simulink model "SpringModel"  (R2018a)
settings: Solver=ode45  StartTime=0.0  StopTime=1  MaxStep=1e-4  MinStep=1e-6  RelTol=1e-4  AbsTol=1e-7
settings Model: Creator=thoma_000  LastModifiedBy=thoma_000
settings SolverCC: ZeroCrossAlgorithm=Adaptive
settings DebuggingCC: MaxConsecutiveZCsMsg=none

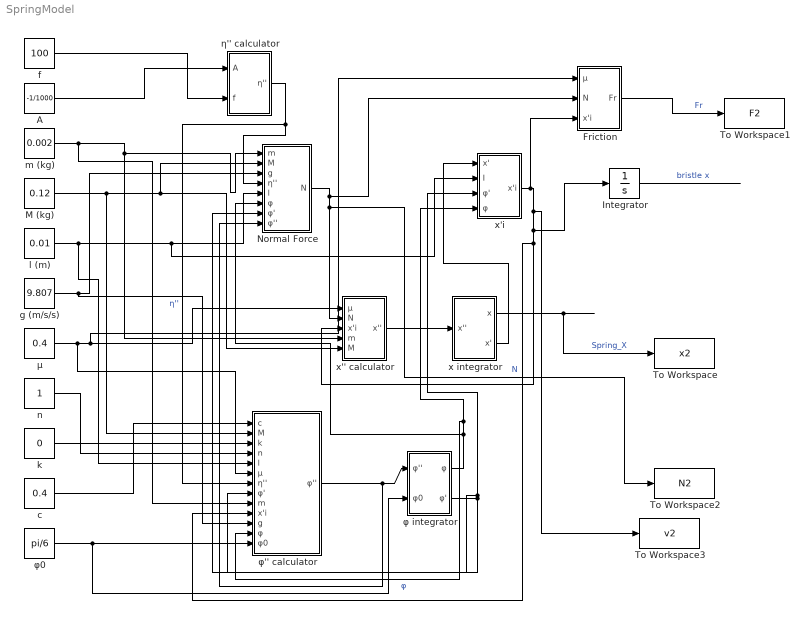
== system SpringModel ==
  A : Constant  Value=-1/1000
  Friction : Subsystem
  Integrator : Integrator
  M (kg) : Constant  Value=0.12
  Normal Force : Subsystem
  To Workspace : ToWorkspace  VariableName=x2  SaveFormat=Timeseries  SampleTime=-1
      settings: Decimation=10
  To Workspace1 : ToWorkspace  VariableName=F2  SaveFormat=Timeseries  SampleTime=-1
      settings: Decimation=10
  To Workspace2 : ToWorkspace  VariableName=N2  SaveFormat=Timeseries  SampleTime=-1
      settings: Decimation=10
  To Workspace3 : ToWorkspace  VariableName=v2  SaveFormat=Timeseries  SampleTime=-1
      settings: Decimation=10
  c : Constant  Value=0.4
  f : Constant  Value=100
  g (m/s/s) : Constant  Value=9.807
  k : Constant  Value=0
  l (m) : Constant  Value=0.01
  m (kg) : Constant  Value=0.002
  n : Constant
  x integrator : Subsystem
  x'' calculator : Subsystem
  x'i : Subsystem
  η'' calculator : Subsystem
  μ : Constant  Value=0.4
  φ integrator : Subsystem
  φ'' calculator : Subsystem
  φ0 : Constant  Value=pi/6
  wires:
  Normal Force/1(N) -> Friction/2(N), To Workspace2/1, x'' calculator/2(N)  "N"
  μ/1 -> φ'' calculator/6(μ), Friction/1(μ), x'' calculator/1(μ)
  x'i/1(x'i) -> Friction/3(x'i), To Workspace3/1, Integrator/1, φ'' calculator/10(x'i), x'' calculator/3(x'i)
  m (kg)/1 -> φ'' calculator/9(m), Normal Force/1(m), x'' calculator/4(m)
  M (kg)/1 -> φ'' calculator/2(M), Normal Force/2(M), x'' calculator/5(M)
  g (m/s/s)/1 -> φ'' calculator/11(g), Normal Force/3(g)
  l (m)/1 -> φ'' calculator/5(l), x'i/2(I), Normal Force/5(l)
  x'' calculator/1(x'') -> x integrator/1(x'')
  x integrator/2(x') -> x'i/1(x')
  x integrator/1(x) -> To Workspace/1  "Spring_X"
  A/1 -> η'' calculator/1(A)
  f/1 -> η'' calculator/2(f)
  η'' calculator/1(η'') -> φ'' calculator/7(η''), Normal Force/4(η'')  "η''"
  φ'' calculator/1(φ'') -> Normal Force/8(φ''), φ integrator/1(φ'')
  φ integrator/1(φ) -> Normal Force/6(φ), φ'' calculator/12(φ), x'i/4(φ)  "φ"
  φ integrator/2(φ') -> x'i/3(φ'), Normal Force/7(φ'), φ'' calculator/8(φ')
  c/1 -> φ'' calculator/1(c)
  k/1 -> φ'' calculator/3(k)
  n/1 -> φ'' calculator/4(n)
  φ0/1 -> φ integrator/2(φ0), φ'' calculator/13(φ0)
  Integrator/1 -> ?  "bristle x"
  Friction/1(Fr) -> To Workspace1/1  "Fr"

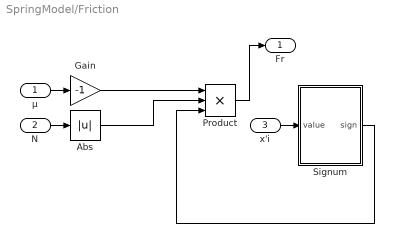
== system SpringModel/Friction ==
  μ : Inport
  N : Inport  Port=2
  x'i : Inport  Port=3
  Abs : Abs
  Gain : Gain  Gain=-1
  Product : Product  Inputs=3
  Signum : Subsystem
  Fr : Outport
  wires:
  Abs/1 -> Product/2
  N/1 -> Abs/1
  Gain/1 -> Product/1
  Signum/1(sign) -> Product/3
  μ/1 -> Gain/1
  Product/1 -> Fr/1
  x'i/1 -> Signum/1(value)

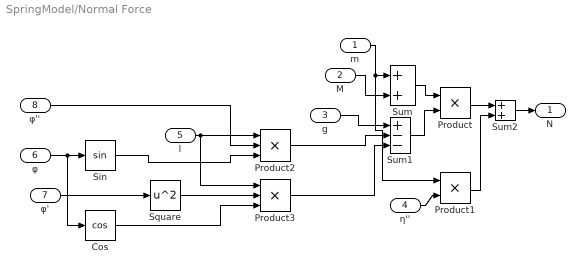
== system SpringModel/Normal Force ==
  m : Inport
  M : Inport  Port=2
  g : Inport  Port=3
  η'' : Inport  Port=4
  l : Inport  Port=5
  φ : Inport  Port=6
  φ' : Inport  Port=7
  φ'' : Inport  Port=8
  Cos : Trigonometry  Operator=cos
  Product : Product
  Product1 : Product
  Product2 : Product  Inputs=***
  Product3 : Product  Inputs=***
  Sin : Trigonometry
  Square : Math  Operator=square  SaturateOnIntegerOverflow=on
  Sum : Sum
  Sum1 : Sum  Inputs=+--
  Sum2 : Sum
  N : Outport
  wires:
  Sum1/1 -> Product/2
  Sum2/1 -> N/1
  Product/1 -> Sum2/1
  η''/1 -> Product1/2
  Product2/1 -> Sum1/2
  Sum/1 -> Product/1
  Product3/1 -> Sum1/3
  Product1/1 -> Sum2/2
  g/1 -> Sum1/1
  m/1 -> Product1/1, Sum/1
  M/1 -> Sum/2
  l/1 -> Product3/1, Product2/1
  Square/1 -> Product3/2
  Sin/1 -> Product2/3
  Cos/1 -> Product3/3
  φ/1 -> Sin/1, Cos/1
  φ'/1 -> Square/1
  φ''/1 -> Product2/2

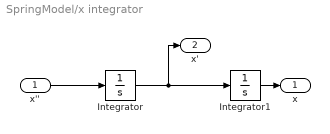
== system SpringModel/x integrator ==
  x'' : Inport
  Integrator : Integrator
  Integrator1 : Integrator
  x : Outport
  x' : Outport  Port=2
  wires:
  Integrator/1 -> x'/1, Integrator1/1
  Integrator1/1 -> x/1
  x''/1 -> Integrator/1

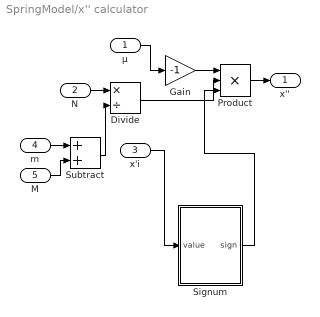
== system SpringModel/x'' calculator ==
  μ : Inport
  N : Inport  Port=2
  x'i : Inport  Port=3
  m : Inport  Port=4
  M : Inport  Port=5
  Divide : Product  Inputs=*/
  Gain : Gain  Gain=-1
  Product : Product  Inputs=***
  Signum : Subsystem
  Subtract : Sum
  x'' : Outport
  wires:
  N/1 -> Divide/1
  M/1 -> Subtract/2
  Subtract/1 -> Divide/2
  Signum/1(sign) -> Product/3
  μ/1 -> Gain/1
  Divide/1 -> Product/2
  m/1 -> Subtract/1
  Gain/1 -> Product/1
  x'i/1 -> Signum/1(value)
  Product/1 -> x''/1

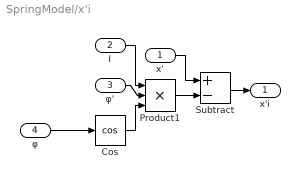
== system SpringModel/x'i ==
  x' : Inport
  I : Inport  Port=2
  φ' : Inport  Port=3
  φ : Inport  Port=4
  Cos : Trigonometry  Operator=cos
  Product1 : Product  Inputs=***
  Subtract : Sum  Inputs=+-
  x'i : Outport
  wires:
  x'/1 -> Subtract/1
  φ/1 -> Cos/1
  Product1/1 -> Subtract/2
  Cos/1 -> Product1/3
  I/1 -> Product1/1
  φ'/1 -> Product1/2
  Subtract/1 -> x'i/1

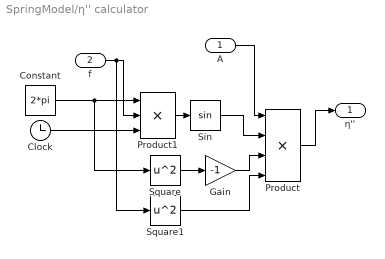
== system SpringModel/η'' calculator ==
  A : Inport
  f : Inport  Port=2
  Clock : Clock
  Constant : Constant  Value=2*pi
  Gain : Gain  Gain=-1
  Product : Product  Inputs=4
  Product1 : Product  Inputs=***
  Sin : Trigonometry
  Square : Math  Operator=square  SaturateOnIntegerOverflow=on
  Square1 : Math  Operator=square  SaturateOnIntegerOverflow=on
  η'' : Outport
  wires:
  Product1/1 -> Sin/1
  A/1 -> Product/1
  Sin/1 -> Product/2
  Clock/1 -> Product1/3
  Constant/1 -> Square/1, Product1/1
  Product/1 -> η''/1
  f/1 -> Square1/1, Product1/2
  Square/1 -> Gain/1
  Gain/1 -> Product/3
  Square1/1 -> Product/4

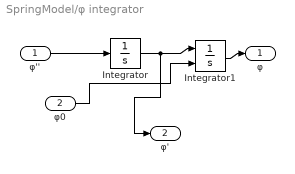
== system SpringModel/φ integrator ==
  φ'' : Inport
  φ0 : Inport  Port=2
  Integrator : Integrator
  Integrator1 : Integrator  InitialConditionSource=external  InitialCondition=pi/6
  φ : Outport
  φ' : Outport  Port=2
  wires:
  φ''/1 -> Integrator/1
  Integrator/1 -> φ'/1, Integrator1/1
  Integrator1/1 -> φ/1
  φ0/1 -> Integrator1/2

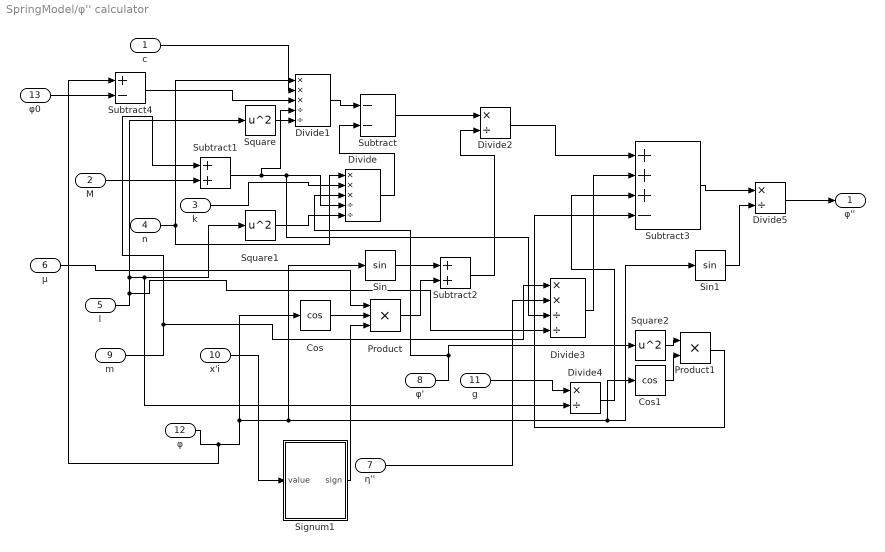
== system SpringModel/φ'' calculator ==
  c : Inport
  M : Inport  Port=2
  k : Inport  Port=3
  n : Inport  Port=4
  l : Inport  Port=5
  μ : Inport  Port=6
  η'' : Inport  Port=7
  φ' : Inport  Port=8
  m : Inport  Port=9
  x'i : Inport  Port=10
  g : Inport  Port=11
  φ : Inport  Port=12
  φ0 : Inport  Port=13
  Cos : Trigonometry  Operator=cos
  Cos1 : Trigonometry  Operator=cos
  Divide : Product  Inputs=***//
  Divide1 : Product  Inputs=***//
  Divide2 : Product  Inputs=*/
  Divide3 : Product  Inputs=**//
  Divide4 : Product  Inputs=*/
  Divide5 : Product  Inputs=*/
  Product : Product  Inputs=***
  Product1 : Product
  Signum1 : Subsystem
  Sin : Trigonometry
  Sin1 : Trigonometry
  Square : Math  Operator=square  SaturateOnIntegerOverflow=on
  Square1 : Math  Operator=square  SaturateOnIntegerOverflow=on
  Square2 : Math  Operator=square  SaturateOnIntegerOverflow=on
  Subtract : Sum  Inputs=--
  Subtract1 : Sum
  Subtract2 : Sum
  Subtract3 : Sum  Inputs=+++-
  Subtract4 : Sum  Inputs=+-
  φ'' : Outport
  wires:
  Signum1/1(sign) -> Product/3
  m/1 -> Divide3/1, Subtract1/1
  Product1/1 -> Subtract3/4
  Subtract1/1 -> Divide1/4, Divide3/3, Divide/4
  l/1 -> Divide3/4, Divide4/2, Square1/1, Square/1
  M/1 -> Subtract1/2
  Divide5/1 -> φ''/1
  Divide3/1 -> Subtract3/2
  x'i/1 -> Signum1/1(value)
  Square/1 -> Divide1/5
  Square1/1 -> Divide/5
  φ/1 -> Subtract4/1, Cos/1, Cos1/1, Sin1/1, Sin/1
  n/1 -> Divide1/1, Divide/1
  Cos/1 -> Product/2
  c/1 -> Divide1/2
  Product/1 -> Subtract2/2
  μ/1 -> Product/1
  Subtract/1 -> Divide2/1
  Divide4/1 -> Subtract3/3
  Cos1/1 -> Product1/2
  φ'/1 -> Divide/3, Square2/1
  Divide/1 -> Subtract/2
  Divide1/1 -> Subtract/1
  Square2/1 -> Product1/1
  Sin1/1 -> Divide5/2
  Subtract3/1 -> Divide5/1
  Sin/1 -> Subtract2/1
  Subtract2/1 -> Divide2/2
  g/1 -> Divide4/1
  Divide2/1 -> Subtract3/1
  k/1 -> Divide/2
  η''/1 -> Divide3/2
  Subtract4/1 -> Divide1/3
  φ0/1 -> Subtract4/2

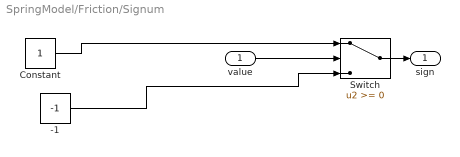
== system SpringModel/Friction/Signum ==
  value : Inport
  -1 : Constant  Value=-1
  Constant : Constant
  Switch : Switch
  sign : Outport
  wires:
  -1/1 -> Switch/3
  Constant/1 -> Switch/1
  Switch/1 -> sign/1
  value/1 -> Switch/2

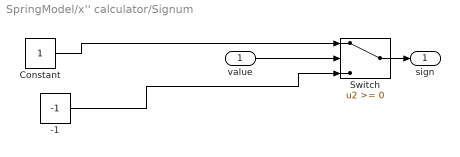
== system SpringModel/x'' calculator/Signum ==
  value : Inport
  -1 : Constant  Value=-1
  Constant : Constant
  Switch : Switch
  sign : Outport
  wires:
  -1/1 -> Switch/3
  Constant/1 -> Switch/1
  Switch/1 -> sign/1
  value/1 -> Switch/2

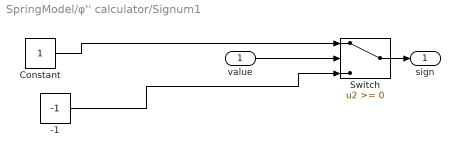
== system SpringModel/φ'' calculator/Signum1 ==
  value : Inport
  -1 : Constant  Value=-1
  Constant : Constant
  Switch : Switch
  sign : Outport
  wires:
  -1/1 -> Switch/3
  Constant/1 -> Switch/1
  Switch/1 -> sign/1
  value/1 -> Switch/2
